simulink model "FSM_Thermostat"  (R2025b)
settings: Solver=VariableStepAuto  StartTime=0.0  StopTime=100  RelTol=1e-3
undefined symbols (not defined in the file): FC, SOC, TC, TD
settings Model: Creator=Tienna Mensah  LastModifiedBy=Tienna Mensah

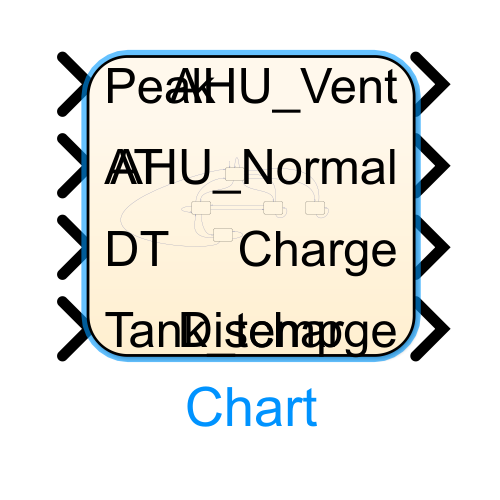
[thumbnail: Simulink's stored preview of the top-level diagram]
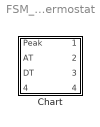
== system FSM_Thermostat ==
  Chart : Stateflow chart  TreatAsAtomicUnit=on

== stateflow chart FSM_Thermostat/Chart ==
  state Idle
    AHU_Vent = ON;
  state AHU_Normal_ON
    AHU_Normal = ON;
    AHU_Vent = ON;
  state Discharge_ON
    Discharge = ON;
    AHU_Vent = ON;
  state Charge_vent
    Charge = ON;
    AHU_Vent = ON;
  state Charge_norm
    Charge = ON;
    AHU_Normal = ON;
  Idle -> Idle [order 4] : [AT >= DT && SOC == FC]
  (default) -> Idle
  Charge_vent -> Idle [order 1] : [Tank_temp >= TC || Peak == 1]
  Charge_norm -> Idle [order 1] : [(Tank_temp >= TC ||Peak ==1) && AT >= DT]
  Discharge_ON -> Idle [order 2] : [AT >= DT]
  AHU_Normal_ON -> Idle [order 2] : [AT >= DT]
  Idle -> Charge_vent [order 1] : [Tank_temp < TC && DT <= AT && Peak == 0]
  Idle -> AHU_Normal_ON [order 2] : [AT < DT && SOC == FC && Peak == 0]
  Idle -> Discharge_ON [order 3] : [AT < DT && Tank_temp >= TC && Peak == 1]
  Discharge_ON -> AHU_Normal_ON [order 1] : [AT < DT && Tank_temp < TD]
  AHU_Normal_ON -> AHU_Normal_ON [order 4] : [[AT < DT && SOC == FC && Peak == 0]]
  Discharge_ON -> Discharge_ON [order 3] : [AT < DT && Tank_temp >= TC && Peak == 1]
  Charge_vent -> Charge_vent [order 2] : [Tank_temp < TC && DT <= AT && Peak == 0]
  AHU_Normal_ON -> Discharge_ON [order 1] : [AT < DT && Tank_temp >= TD && Peak ==1]
  Charge_norm -> AHU_Normal_ON [order 2] : [(Tank_temp >= TC || Peak == 1) && AT < DT]
  AHU_Normal_ON -> Charge_norm [order 3] : [Tank_temp < TD && Peak == 0]
  Charge_norm -> Charge_norm [order 3] : [Tank_temp < TD && Peak == 0]
  data: Peak input; AHU_Vent output; AHU_Normal output; ON parameter; AT input; SOC parameter; DT input; FC parameter; Charge output; Discharge output; TC parameter; TD parameter; Tank_temp input
